simulink model "bacteria"  (R2023b)
settings: Solver=VariableStepAuto  StartTime=0.0  StopTime=10.0  RelTol=1e-3
settings Model: Creator=allonso77  LastModifiedBy=allonso77

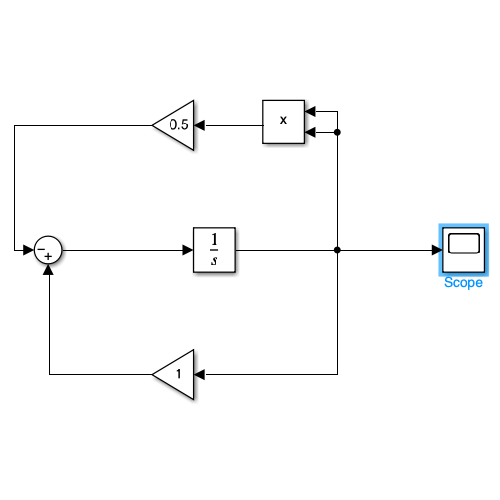
[thumbnail: Simulink's stored preview of the top-level diagram]
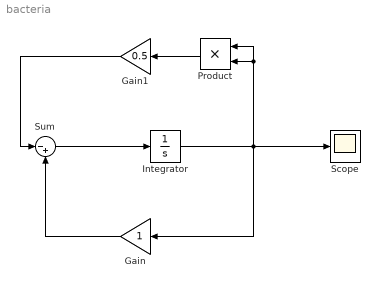
== system bacteria ==
  Gain : Gain
  Gain1 : Gain  Gain=0.5
  Integrator : Integrator  InitialCondition=100
  Product : Product
  Scope : Scope
  Sum : Sum  Inputs=|-+
  wires:
  Sum/1 -> Integrator/1
  Integrator/1 -> Gain/1, Product/2, Product/1, Scope/1
  Gain/1 -> Sum/2
  Gain1/1 -> Sum/1
  Product/1 -> Gain1/1
